simulink model "lookuptableR17a"  (R2017a)
settings: Solver=FixedStepAuto  StartTime=0.0  StopTime=tf  FixedStep=0.001  RelTol=1e-3
libraries: simulink x1
settings Model: Creator=Home  LastModifiedBy=Home

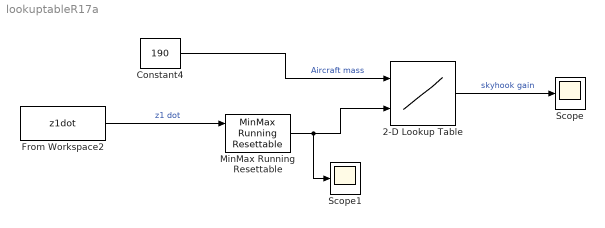
== system lookuptableR17a ==
  2-D Lookup Table : Lookup_n-D  BreakpointsForDimension1=[0,150,190,230]  BreakpointsForDimension2=[0,1,2,3,4]  Table=reshape([0,0,300,700,0,0,300,700,0,0,0,300,0,0,0,100,0,0,0,100],4,5)  InternalRulePriority=Speed  RndMeth=Simplest  InputSameDT=on
  Constant4 : Constant  Value=190
  From Workspace2 : FromWorkspace  VariableName=z1dot  SampleTime=0
  MinMax Running Resettable : simulink/Math Operations/MinMax Running Resettable  Function=max  vinit=0.0
  Scope : Scope
  Scope1 : Scope
  wires:
  From Workspace2/1 -> MinMax Running Resettable/1  "z1 dot"
  MinMax Running Resettable/1 -> Scope1/1, 2-D Lookup Table/2
  Constant4/1 -> 2-D Lookup Table/1  "Aircraft mass"
  2-D Lookup Table/1 -> Scope/1  "skyhook gain"
